simulink model "Arrays1"  (Simulink 8.7)
settings: Solver=FixedStepDiscrete  StartTime=0.0  StopTime=10000.0  RelTol=1e-3
settings Model: Creator=scaife  LastModifiedBy=bourbouh  ExtModeAutoUpdateStatusClock=off
settings DataIOCC: SignalLoggingSaveFormat=ModelDataLogs  SignalLoggingName=sigsOut
settings DebuggingCC: SaveWithParameterizedLinksMsg=none  SignalResolutionControl=TryResolveAllWithWarning  MultiTaskDSMMsg=warning  MultiTaskCondExecSysMsg=none  StrictBusMsg=None
settings HardwareCC: TargetUnknown=on
settings SFSimCC: SimParseCustomCode=off
settings GRTTargetCC: CombineOutputUpdateFcns=off  GRTInterface=on

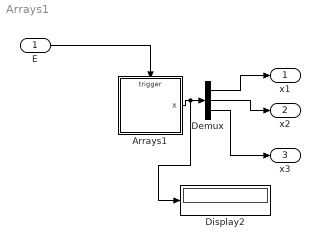
== system Arrays1 ==
  E : Inport
  Arrays1 : Stateflow chart  TreatAsAtomicUnit=on
  Demux : Demux  Outputs=3
  Display2 : Display
  x1 : Outport
  x2 : Outport  Port=2
  x3 : Outport  Port=3
  wires:
  E/1 -> Arrays1/Trigger
  Arrays1/1(x) -> Display2/1, Demux/1
  Demux/1 -> x1/1
  Demux/2 -> x2/1
  Demux/3 -> x3/1

== stateflow chart Arrays1 ==
  state A/
    en:x[1]++;
  state B/
    en:x[2]++;
  state C/
    en:x[3]++;
  (default) -> A
  A -> B : E
  C -> A : E
  B -> C : E
  data: x output int32 size=3 [0..100] =1
  events: E input RISING_EDGE_EVENT
